simulink library "STATE_BIO_MASTER"  (Simulink 8.6)
settings: Solver=ode45  StartTime=0.0  StopTime=10.0  RelTol=1e-3
libraries: cdsBitwise x48, cdsEpicsIn x41, cdsFunctionCall x10, cdsEpicsOut x7
(part 2 of 2)

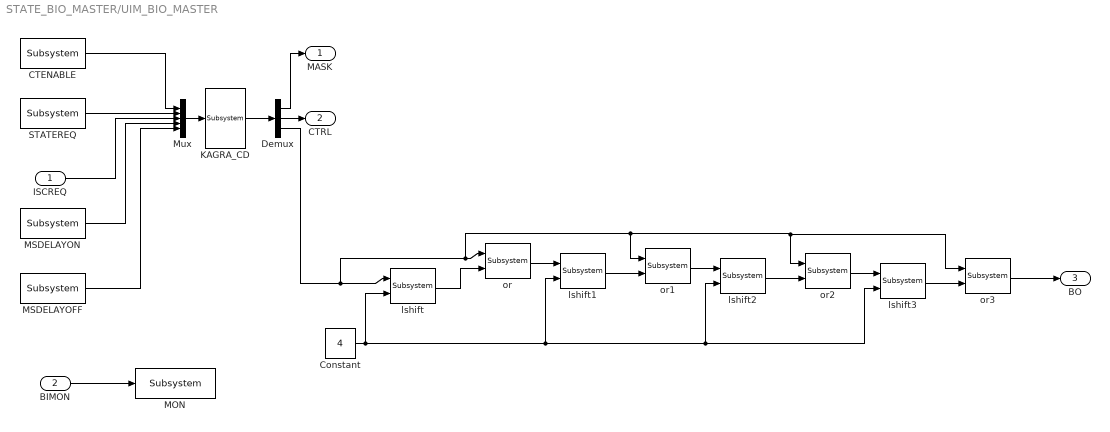
== system STATE_BIO_MASTER/UIM_BIO_MASTER ==
  ISCREQ : Inport
  BIMON : Inport  Port=2
  CTENABLE : cdsEpicsIn/Subsystem  Tag=cdsEpicsIn  Description=|
      | Purpose:                                                                              
      | Create an EPICS input channel connection to the FE realtime controls.                 
      |                                                                                       
      | Operation:                                                                            
      | Outputs value from an EPICS ai record. Value is floating point with a precision of 3..
      |                                                                                       
      | Usage:                                                                                
      | Name the part with the desired EPICS channel name.
      settings: AttributesFormatString=%<Tag>
  Constant : Constant  Value=4
  Demux : Demux  Outputs=3
  KAGRA_CD : cdsFunctionCall/Subsystem  Tag=cdsFunctionCall  Description=inline KAGRA_CD /opt/rtcds/userapps/trunk/vis/common/src/CD_STATE_MACHINE_KAGRA.c
      settings: AttributesFormatString=%<Tag>
  MON : cdsEpicsOut/Subsystem  Tag=cdsEpicsOutput  Description=|
      | Purpose:                                          
      | Output a FE signal to an EPICS channel.           
      |                                                   
      | Operation:                                        
      | Takes input value and passes it to EPICS record.  
      |                                                   
      | Usage:                                            
      | Name the part with the desired EPICS rrecord name.
      settings: AttributesFormatString=%<Tag>
  MSDELAYOFF : cdsEpicsIn/Subsystem  Tag=cdsEpicsIn  Description=|
      | Purpose:                                                                              
      | Create an EPICS input channel connection to the FE realtime controls.                 
      |                                                                                       
      | Operation:                                                                            
      | Outputs value from an EPICS ai record. Value is floating point with a precision of 3..
      |                                                                                       
      | Usage:                                                                                
      | Name the part with the desired EPICS channel name.
      settings: AttributesFormatString=%<Tag>
  MSDELAYON : cdsEpicsIn/Subsystem  Tag=cdsEpicsIn  Description=|
      | Purpose:                                                                              
      | Create an EPICS input channel connection to the FE realtime controls.                 
      |                                                                                       
      | Operation:                                                                            
      | Outputs value from an EPICS ai record. Value is floating point with a precision of 3..
      |                                                                                       
      | Usage:                                                                                
      | Name the part with the desired EPICS channel name.
      settings: AttributesFormatString=%<Tag>
  Mux : Mux  Inputs=5
  STATEREQ : cdsEpicsIn/Subsystem  Tag=cdsEpicsIn  Description=|
      | Purpose:                                                                              
      | Create an EPICS input channel connection to the FE realtime controls.                 
      |                                                                                       
      | Operation:                                                                            
      | Outputs value from an EPICS ai record. Value is floating point with a precision of 3..
      |                                                                                       
      | Usage:                                                                                
      | Name the part with the desired EPICS channel name.
      settings: AttributesFormatString=%<Tag>
  lshift{,1..3} (4 alike) : cdsBitwise/Subsystem  Tag=cdsBitwise
      settings: AttributesFormatString=%<Tag>
  or{,1..3} (4 alike) : cdsBitwise/Subsystem  Tag=cdsBitwise
      settings: AttributesFormatString=%<Tag>
  MASK : Outport
  CTRL : Outport  Port=2
  BO : Outport  Port=3
  wires:
  Demux/3 -> or3/1, or2/1, or1/1, or/1, lshift/1
  lshift2/1 -> or2/2
  or1/1 -> lshift2/1
  lshift1/1 -> or1/2
  or/1 -> lshift1/1
  lshift/1 -> or/2
  MSDELAYOFF/1 -> Mux/5
  KAGRA_CD/1 -> Demux/1
  Mux/1 -> KAGRA_CD/1
  CTENABLE/1 -> Mux/1
  STATEREQ/1 -> Mux/2
  ISCREQ/1 -> Mux/3
  MSDELAYON/1 -> Mux/4
  Demux/1 -> MASK/1
  Demux/2 -> CTRL/1
  BIMON/1 -> MON/1
  or2/1 -> lshift3/1
  lshift3/1 -> or3/2
  Constant/1 -> lshift2/2, lshift3/2, lshift1/2, lshift/2
  or3/1 -> BO/1
